simulink model "SimulinkModel"  (R2019b)
settings: Solver=VariableStepAuto  StartTime=0.0  StopTime=50000  RelTol=1e-7
settings Model: Creator=Jad Yahya  LastModifiedBy=Jad Yahya

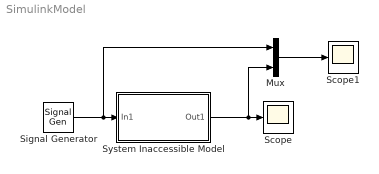
== system SimulinkModel ==
  Mux : Mux  Inputs=2
  Scope : Scope
  Scope1 : Scope
  Signal Generator : SignalGenerator  Units=rad/sec
  System Inaccessible Model : Subsystem
  wires:
  System Inaccessible Model/1(Out1) -> Mux/2, Scope/1
  Signal Generator/1 -> Mux/1, System Inaccessible Model/1(In1)
  Mux/1 -> Scope1/1

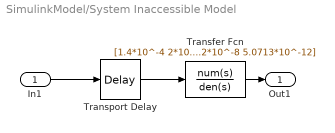
== system SimulinkModel/System Inaccessible Model ==
  In1 : Inport
  Transfer Fcn : TransferFcn  Numerator=[1.4*10^-4 2*10^-7 7.56*10^-12]  Denominator=[1 3.68*10^-2 2.35752*10^-4 8.2*10^-8 5.0713*10^-12]
  Transport Delay : TransportDelay  DelayTime=8.5
  Out1 : Outport
  wires:
  In1/1 -> Transport Delay/1
  Transport Delay/1 -> Transfer Fcn/1
  Transfer Fcn/1 -> Out1/1
